simulink model "vectobin"  (R2020a)
settings: Solver=VariableStepAuto  StartTime=0.0  StopTime=10  RelTol=1e-3
model workspace (MAT data in the model file):
  a = Simulink.Parameter
  a.Value = [1 0 1]
  a.DataType = 'auto'
  a.Dimensions = [1 3]
  ab = [1 1]
settings Model: Creator=F1  LastModifiedBy=F1

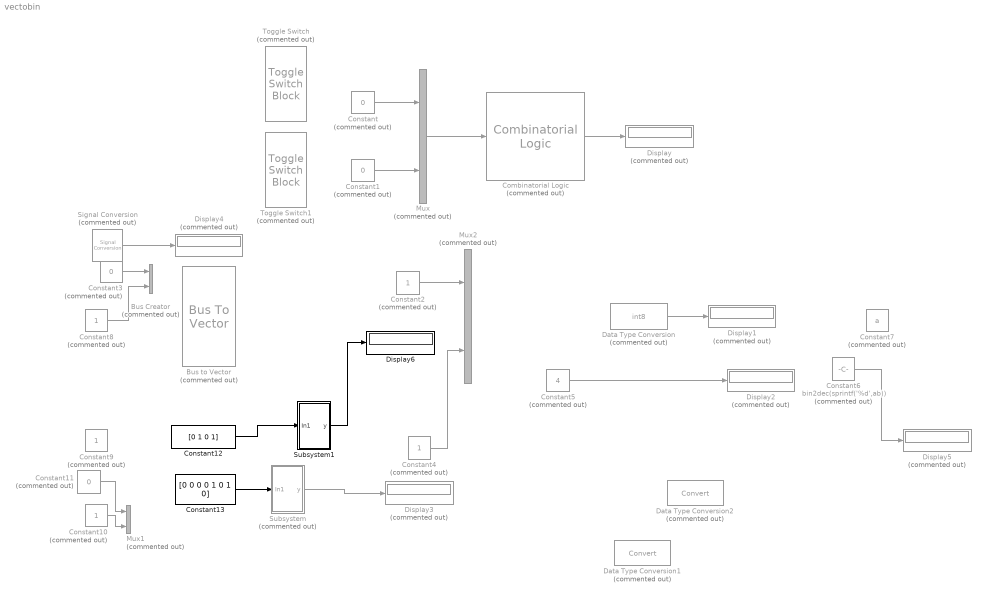
== system vectobin ==
  Bus Creator : BusCreator  Commented=on  Inputs=2
  Bus to Vector : BusToVector  Commented=on
  Combinatorial Logic : CombinatorialLogic  Commented=on  TruthTable=[0;1;1;0]
  Constant{,1,3,11} (4 alike) : Constant  Commented=on  Value=0
  Constant{2,4,8..10} (5 alike) : Constant  Commented=on
  Constant12 : Constant  Value=[0 1 0 1]
  Constant13 : Constant  Value=[0 0 0 0 1 0 1 0]
  Constant5 : Constant  Commented=on  Value=4
  Constant6 : Constant  Commented=on  Value=bin2dec(sprintf('%d',ab))
  Constant7 : Constant  Commented=on  Value=a
  Data Type Conversion : DataTypeConversion  Commented=on  OutMin=[2]  OutDataTypeStr=int8
  Data Type Conversion1 : DataTypeConversion  Commented=on
  Data Type Conversion2 : DataTypeConversion  Commented=on
  Display{,1..5} (6 alike) : Display  Commented=on
      Display2 settings: Format=binary (Stored Integer)
      Display4 settings: Format=decimal (Stored Integer)
  Display6 : Display
  Mux : Mux  Commented=on  Inputs=2
  Mux1 : Mux  Commented=on  Inputs=2
  Mux2 : Mux  Commented=on  Inputs=2
  Signal Conversion : SignalConversion  Commented=on  ConversionOutput=Virtual bus  OverrideOpt=off
  Subsystem : Subsystem  Commented=on
  Subsystem1 : Subsystem
  Toggle Switch : ToggleSwitchBlock  Commented=on
      settings: Values={{'Off', 'On'}, [0 1]}
  Toggle Switch1 : ToggleSwitchBlock  Commented=on
      settings: Values={{'Off', 'On'}, [0 1]}
  wires:
  Constant/1 -> Mux/1
  Constant1/1 -> Mux/2
  Mux/1 -> Combinatorial Logic/1
  Combinatorial Logic/1 -> Display/1
  Data Type Conversion/1 -> Display1/1
  Constant2/1 -> Mux2/1
  Constant4/1 -> Mux2/2
  Constant5/1 -> Display2/1
  Constant6/1 -> Display5/1
  Constant3/1 -> Bus Creator/1
  Constant8/1 -> Bus Creator/2
  Signal Conversion/1 -> Display4/1
  Constant11/1 -> Mux1/1
  Constant10/1 -> Mux1/2
  Constant12/1 -> Subsystem1/1(In1)
  Subsystem/1(y) -> Display3/1
  Subsystem1/1(y) -> Display6/1
  Constant13/1 -> Subsystem/1(In1)

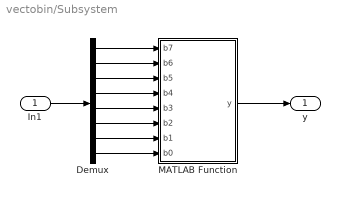
== system vectobin/Subsystem ==
  In1 : Inport
  Demux : Demux  Outputs=8
  MATLAB Function : MATLAB Function  TreatAsAtomicUnit=on
  y : Outport
  wires:
  Demux/8 -> MATLAB Function/8(b0)
  Demux/2 -> MATLAB Function/2(b6)
  MATLAB Function/1(y) -> y/1
  Demux/7 -> MATLAB Function/7(b1)
  Demux/4 -> MATLAB Function/4(b4)
  Demux/6 -> MATLAB Function/6(b2)
  Demux/3 -> MATLAB Function/3(b5)
  Demux/1 -> MATLAB Function/1(b7)
  Demux/5 -> MATLAB Function/5(b3)
  In1/1 -> Demux/1

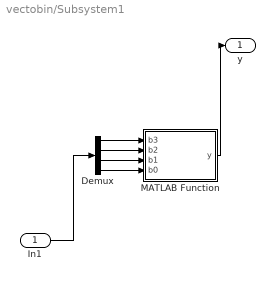
== system vectobin/Subsystem1 ==
  In1 : Inport
  Demux : Demux
  MATLAB Function : MATLAB Function  TreatAsAtomicUnit=on
  y : Outport
  wires:
  Demux/3 -> MATLAB Function/3(b1)
  Demux/1 -> MATLAB Function/1(b3)
  Demux/2 -> MATLAB Function/2(b2)
  Demux/4 -> MATLAB Function/4(b0)
  MATLAB Function/1(y) -> y/1
  In1/1 -> Demux/1

== matlab function vectobin/Subsystem1/MATLAB Function ==
  data: b3 input; y output; b2 input; b1 input; b0 input
function y = fcn( b3   , b2   , b1    , b0    )
y =  b3*2^3 + b2*2^2 + b1*2^1 + b0*2^0 ;
end

== matlab function vectobin/Subsystem/MATLAB Function ==
  data: b7 input; y output [0..255]; b6 input; b5 input; b4 input; b3 input; b2 input; b1 input; b0 input
function y = fcn(b7   , b6  , b5   , b4  , b3   , b2   , b1    , b0    )
y = b7*2^7 + b6*2^6 + b5*2^5 + b4*2^4 + b3*2^3 + b2*2^2 + b1*2^1 + b0*2^0 ;
end



%str_x = sprintf("%i",u);
% remove the spaces in the string, so it 
% becomes '10000000'
%str_x(isspace(str_x)) = '';
% now use BIN2DEC to convert the binary 
% string to a decimal number
%y = bin2dec(str_x);
%y = class(u);
%y = bin2dec(sprintf('%d',u));
